simulink model "RLS"  (R2023a)
settings: Solver=FixedStepAuto  StartTime=start_time  StopTime=stop_time  FixedStep=sample_time  RelTol=1e-3
values from neighbouring files (symbols this model uses):
  A = [1, a]    [example12.m]
  B = b    (= 0.5)    [example12.m]
  C = [1, c]    [example12.m]
  mean_e = 0    [example12.m]    (also in example14.m; example15.m)
  sample_time = 1    [example12.m]    (also in example14.m; example15.m; example16.m)
  seed_e = 6    [example12.m]    (also in example14.m = i; example15.m = 2)
  std_e = 0.5    [example12.m]    (also in example14.m; example15.m)
settings Model: Creator=Beigi  LastModifiedBy=Mmoha

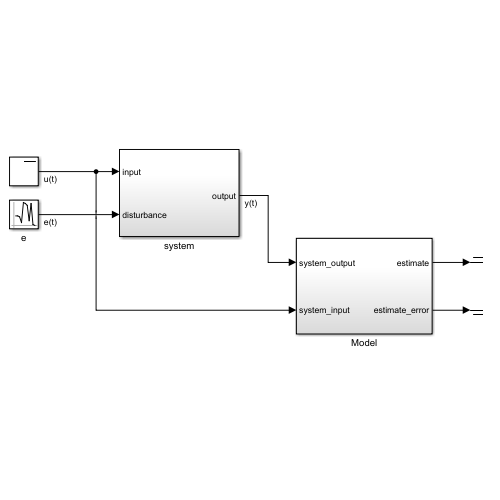
[thumbnail: Simulink's stored preview of the top-level diagram]
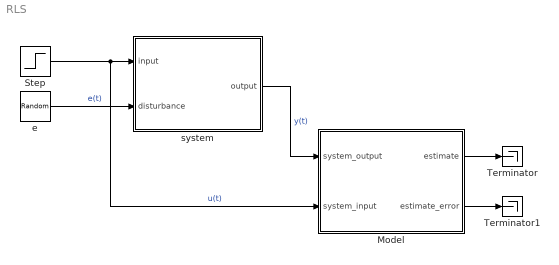
== system RLS ==
  Model : Subsystem
  Step : Step  SampleTime=0
  Terminator : Terminator
  Terminator1 : Terminator
  e : RandomNumber  Mean=mean_e  Variance=std_e^2  Seed=seed_e  SampleTime=sample_time
  system : Subsystem
  wires:
  Model/2(estimate_error) -> Terminator1/1
  Step/1 -> Model/2(system_input), system/1(input)  "u(t)"
  e/1 -> system/2(disturbance)  "e(t)"
  system/1(output) -> Model/1(system_output)  "y(t)"
  Model/1(estimate) -> Terminator/1

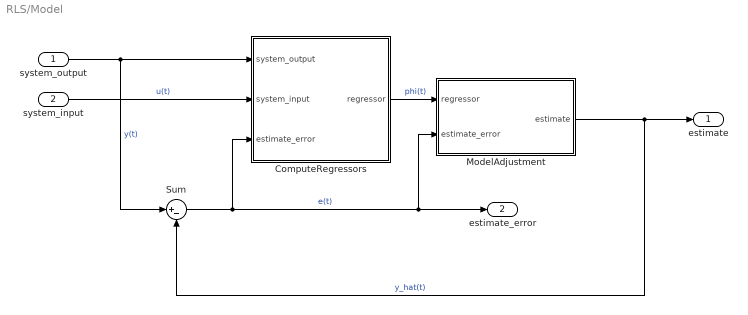
== system RLS/Model ==
  system_output : Inport
  system_input : Inport  Port=2
  ComputeRegressors : Subsystem
  ModelAdjustment : Subsystem
  Sum : Sum  Inputs=|+-
  estimate : Outport
  estimate_error : Outport  Port=2
  wires:
  Sum/1 -> ComputeRegressors/3(estimate_error), ModelAdjustment/2(estimate_error), estimate_error/1  "e(t)"
  system_input/1 -> ComputeRegressors/2(system_input)  "u(t)"
  system_output/1 -> Sum/1, ComputeRegressors/1(system_output)  "y(t)"
  ComputeRegressors/1(regressor) -> ModelAdjustment/1(regressor)  "phi(t)"
  ModelAdjustment/1(estimate) -> Sum/2, estimate/1  "y_hat(t)"

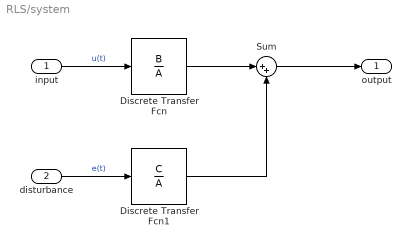
== system RLS/system ==
  input : Inport
  disturbance : Inport  Port=2
  Discrete Transfer Fcn : DiscreteTransferFcn  Numerator=B  Denominator=A
  Discrete Transfer Fcn1 : DiscreteTransferFcn  Numerator=C  Denominator=A
  Sum : Sum  Inputs=|++
  output : Outport
  wires:
  disturbance/1 -> Discrete Transfer Fcn1/1  "e(t)"
  input/1 -> Discrete Transfer Fcn/1  "u(t)"
  Discrete Transfer Fcn/1 -> Sum/1
  Discrete Transfer Fcn1/1 -> Sum/2
  Sum/1 -> output/1

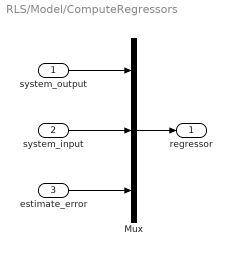
== system RLS/Model/ComputeRegressors ==
  system_output : Inport
  system_input : Inport  Port=2
  estimate_error : Inport  Port=3
  Mux : Mux  Inputs=3
  regressor : Outport
  wires:
  system_output/1 -> Mux/1
  estimate_error/1 -> Mux/3
  system_input/1 -> Mux/2
  Mux/1 -> regressor/1

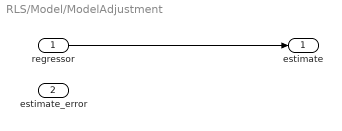
== system RLS/Model/ModelAdjustment ==
  regressor : Inport
  estimate_error : Inport  Port=2
  estimate : Outport
  wires:
  regressor/1 -> estimate/1
